simulink model "Problem4"  (R2020b)
settings: Solver=VariableStepAuto  StartTime=0.0  StopTime=10.0  RelTol=1e-3
settings Model: Creator=Acer  LastModifiedBy=Acer

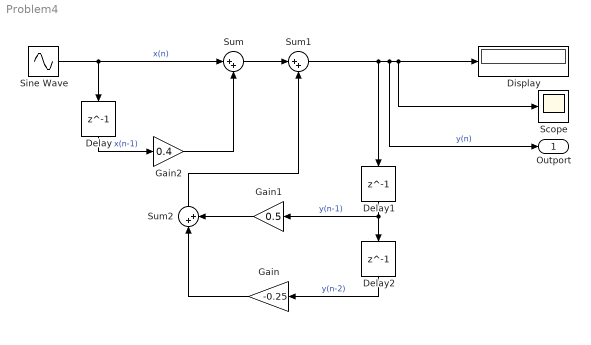
== system Problem4 ==
  Delay : Delay  DelayLength=1
  Delay1 : Delay  DelayLength=1
  Delay2 : Delay  DelayLength=1
  Display : Display
  Gain : Gain  Gain=-0.25
  Gain1 : Gain  Gain=0.5
  Gain2 : Gain  Gain=0.4
  Scope : Scope
  Sine Wave : Sin  SampleTime=0
  Sum : Sum  Inputs=|++
  Sum1 : Sum  Inputs=|++
  Sum2 : Sum  Inputs=|++
  Outport : Outport
  wires:
  Gain/1 -> Sum2/1
  Gain2/1 -> Sum/2
  Sine Wave/1 -> Sum/1, Delay/1  "x(n)"
  Sum/1 -> Sum1/1
  Gain1/1 -> Sum2/2
  Sum2/1 -> Sum1/2
  Delay1/1 -> Delay2/1, Gain1/1  "y(n-1)"
  Delay2/1 -> Gain/1  "y(n-2)"
  Delay/1 -> Gain2/1  "x(n-1)"
  Sum1/1 -> Outport/1, Scope/1, Display/1, Delay1/1  "y(n)"
